simulink model "TST_GbxNPos_DD"  (R2016b)
settings: Solver=FixedStepDiscrete  StartTime=0.0  StopTime=simTime  FixedStep=sampleTime  RelTol=1e-3
values from neighbouring files (symbols this model uses):
  testCase = 1    [initTST_GbxNPos_DD_001.m]
libraries: simulink x3, UnitTest_Lib x1
settings Model: Creator=bianxuyin  LastModifiedBy=bianxuyin
settings DebuggingCC: SignalRangeChecking=error

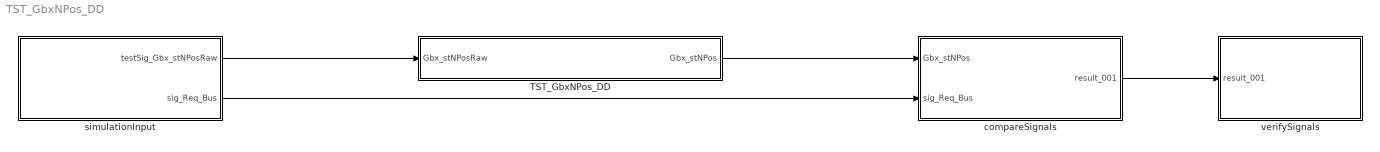
== system TST_GbxNPos_DD ==
  TST_GbxNPos_DD : Subsystem
  compareSignals : Subsystem
  simulationInput : Subsystem
  verifySignals : Subsystem
  wires:
  simulationInput/1(testSig_Gbx_stNPosRaw) -> TST_GbxNPos_DD/1(Gbx_stNPosRaw)
  TST_GbxNPos_DD/1(Gbx_stNPos) -> compareSignals/1(Gbx_stNPos)
  simulationInput/2(sig_Req_Bus) -> compareSignals/2(sig_Req_Bus)
  compareSignals/1(result_001) -> verifySignals/1(result_001)

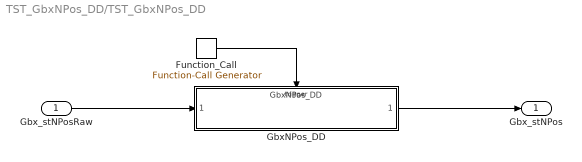
== system TST_GbxNPos_DD/TST_GbxNPos_DD ==
  Gbx_stNPosRaw : Inport
  Function_Call : simulink/Ports & Subsystems/Function-Call Generator  sample_time=sampleTime  numberOfIterations=1
  GbxNPos_DD : ModelReference  ModelNameDialog=GbxNPos_DD  SimulationMode=Normal  ModelReferenceVersion=1.8  TriggerPortName=function  TriggerPortTriggerType=function-call  TriggerPortStatesWhenEnabling=held
  Gbx_stNPos : Outport
  wires:
  Function_Call/1 -> GbxNPos_DD/Trigger
  Gbx_stNPosRaw/1 -> GbxNPos_DD/1
  GbxNPos_DD/1 -> Gbx_stNPos/1

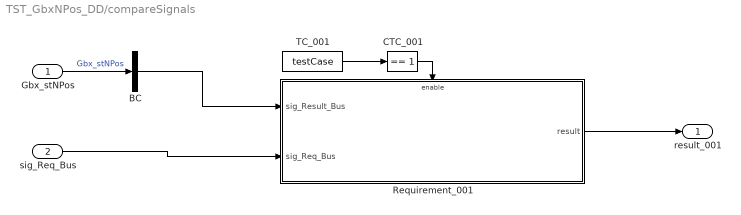
== system TST_GbxNPos_DD/compareSignals ==
  Gbx_stNPos : Inport
  sig_Req_Bus : Inport  Port=2
  BC : BusCreator  Inputs=1
  CTC_001 : simulink/Logic and Bit Operations/Compare To Constant  relop===  const=1  OutDataTypeStr=boolean
  Requirement_001 : Subsystem
  TC_001 : Constant  Value=testCase
  result_001 : Outport
  wires:
  Gbx_stNPos/1 -> BC/1  "Gbx_stNPos"
  TC_001/1 -> CTC_001/1
  CTC_001/1 -> Requirement_001/Enable
  sig_Req_Bus/1 -> Requirement_001/2(sig_Req_Bus)
  BC/1 -> Requirement_001/1(sig_Result_Bus)
  Requirement_001/1(result) -> result_001/1

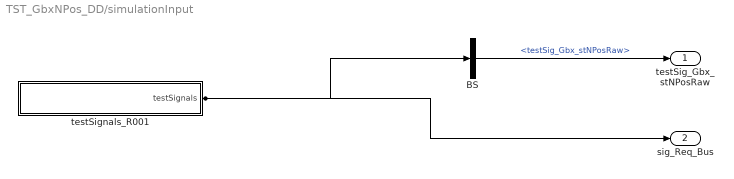
== system TST_GbxNPos_DD/simulationInput ==
  BS : BusSelector  OutputSignals=testSig_Gbx_stNPosRaw
  testSignals_R001 : Subsystem
  testSig_Gbx_stNPosRaw : Outport
  sig_Req_Bus : Outport  Port=2
  wires:
  BS/1 -> testSig_Gbx_stNPosRaw/1  "<testSig_Gbx_stNPosRaw>"
  testSignals_R001/1(testSignals) -> BS/1, sig_Req_Bus/1

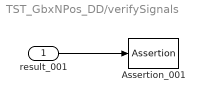
== system TST_GbxNPos_DD/verifySignals ==
  result_001 : Inport
  Assertion_001 : Assertion  Enabled=off
  wires:
  result_001/1 -> Assertion_001/1

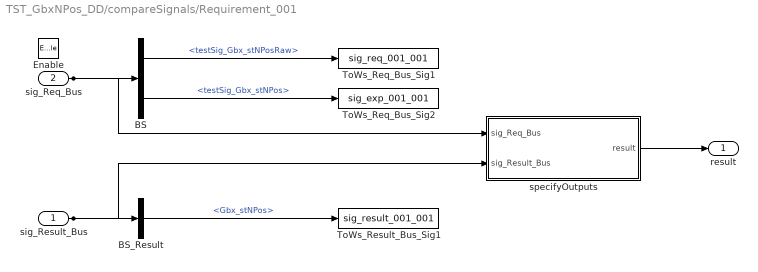
== system TST_GbxNPos_DD/compareSignals/Requirement_001 ==
  sig_Result_Bus : Inport
  sig_Req_Bus : Inport  Port=2
  Enable : EnablePort
  BS : BusSelector  OutputSignals=testSig_Gbx_stNPosRaw,testSig_Gbx_stNPos
  BS_Result : BusSelector  OutputSignals=Gbx_stNPos
  ToWs_Req_Bus_Sig1 : ToWorkspace  VariableName=sig_req_001_001  SaveFormat=Structure With Time
  ToWs_Req_Bus_Sig2 : ToWorkspace  VariableName=sig_exp_001_001  SaveFormat=Structure With Time
  ToWs_Result_Bus_Sig1 : ToWorkspace  VariableName=sig_result_001_001  SaveFormat=Structure With Time
  specifyOutputs : Subsystem
  result : Outport
  wires:
  sig_Req_Bus/1 -> BS/1, specifyOutputs/1(sig_Req_Bus)
  BS/1 -> ToWs_Req_Bus_Sig1/1  "<testSig_Gbx_stNPosRaw>"
  BS/2 -> ToWs_Req_Bus_Sig2/1  "<testSig_Gbx_stNPos>"
  sig_Result_Bus/1 -> BS_Result/1, specifyOutputs/2(sig_Result_Bus)
  BS_Result/1 -> ToWs_Result_Bus_Sig1/1  "<Gbx_stNPos>"
  specifyOutputs/1(result) -> result/1

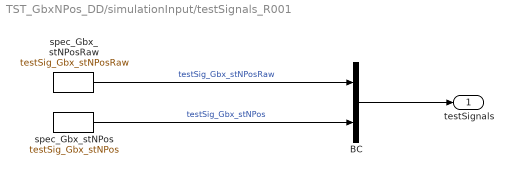
== system TST_GbxNPos_DD/simulationInput/testSignals_R001 ==
  BC : BusCreator  Inputs=2
  spec_Gbx_stNPos : FromWorkspace  VariableName=testSig_Gbx_stNPos  Interpolate=off  OutputAfterFinalValue=Holding final value
  spec_Gbx_stNPosRaw : FromWorkspace  VariableName=testSig_Gbx_stNPosRaw  Interpolate=off  OutputAfterFinalValue=Holding final value
  testSignals : Outport
  wires:
  BC/1 -> testSignals/1
  spec_Gbx_stNPosRaw/1 -> BC/1  "testSig_Gbx_stNPosRaw"
  spec_Gbx_stNPos/1 -> BC/2  "testSig_Gbx_stNPos"

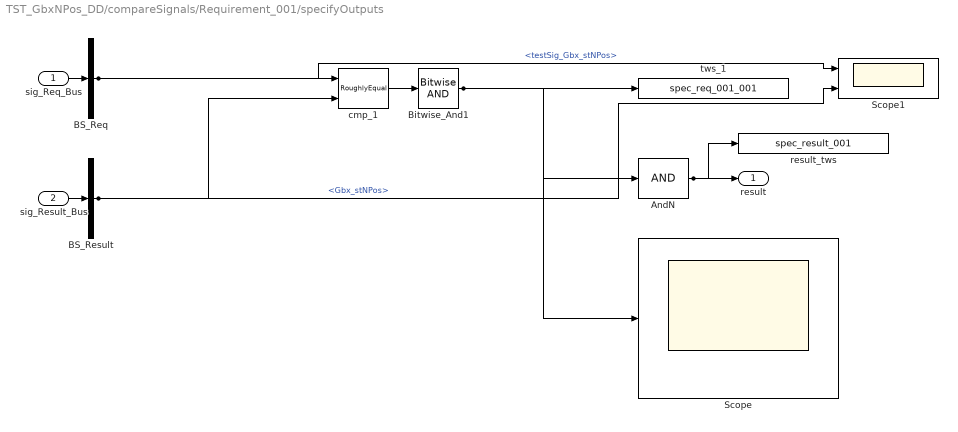
== system TST_GbxNPos_DD/compareSignals/Requirement_001/specifyOutputs ==
  sig_Req_Bus : Inport
  sig_Result_Bus : Inport  Port=2
  AndN : Logic  Inputs=1
  BS_Req : BusSelector  OutputSignals=testSig_Gbx_stNPos
  BS_Result : BusSelector  OutputSignals=Gbx_stNPos
  Bitwise_And1 : simulink/Logic and Bit Operations/Bitwise Operator  logicop=AND  UseBitMask=off  BitMask=bin2dec('11011001')  BitMaskRealWorld=Stored Integer
  Scope : Scope
  Scope1 : Scope  NumInputPorts=2
  cmp_1 : UnitTest_Lib/RoughlyEqual  slope=0.1
  result_tws : ToWorkspace  VariableName=spec_result_001
  tws_1 : ToWorkspace  VariableName=spec_req_001_001
  result : Outport
  wires:
  sig_Req_Bus/1 -> BS_Req/1
  sig_Result_Bus/1 -> BS_Result/1
  AndN/1 -> result/1, result_tws/1
  BS_Req/1 -> cmp_1/1, Scope1/1  "<testSig_Gbx_stNPos>"
  BS_Result/1 -> cmp_1/2, Scope1/2  "<Gbx_stNPos>"
  cmp_1/1 -> Bitwise_And1/1
  Bitwise_And1/1 -> tws_1/1, AndN/1, Scope/1
